simulink model "test_sim"  (R2022b)
settings: Solver=ode4  StartTime=0.0  StopTime=50.0  FixedStep=0.01  RelTol=1e-3
values from neighbouring files (symbols this model uses):
  tau1 = 0.5    [paraset.m]
  tau2 = 2    [paraset.m]
settings Model: Creator=user  LastModifiedBy=user
settings DataIOCC: ReturnWorkspaceOutputs=off

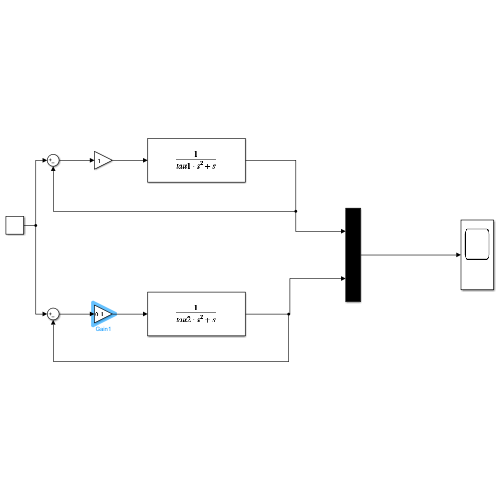
[thumbnail: Simulink's stored preview of the top-level diagram]
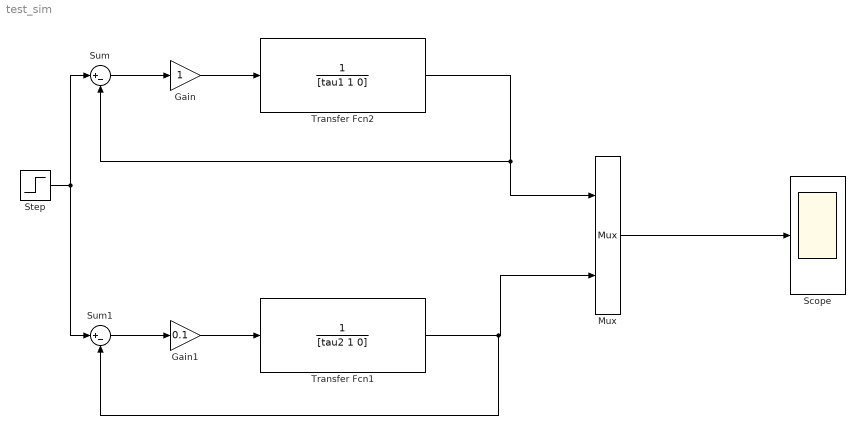
== system test_sim ==
  Gain : Gain
  Gain1 : Gain  Gain=0.1
  Mux : Mux  Inputs=2
  Scope : Scope
  Step : Step  After=100  SampleTime=0
  Sum : Sum  Inputs=|+-
  Sum1 : Sum  Inputs=|+-
  Transfer Fcn1 : TransferFcn  Denominator=[tau2 1 0]
  Transfer Fcn2 : TransferFcn  Denominator=[tau1 1 0]
  wires:
  Transfer Fcn2/1 -> Sum/2, Mux/1
  Transfer Fcn1/1 -> Mux/2, Sum1/2
  Mux/1 -> Scope/1
  Sum/1 -> Gain/1
  Gain/1 -> Transfer Fcn2/1
  Step/1 -> Sum1/1, Sum/1
  Gain1/1 -> Transfer Fcn1/1
  Sum1/1 -> Gain1/1
